simulink model "MAE547Project_part5ModifiedToWorkWithSingularity"  (R2020b)
settings: Solver=VariableStepAuto  StartTime=0.0  StopTime=5  RelTol=1e-3
values from neighbouring files (symbols this model uses):
  Arm = dhfunc(descriptor,d,a,alpha,theta,m,I,r,G,Jm,fv)    [Test.m]    (also in TestZone.m = dhfunc(descriptor,d,a,alpha,theta,m,I,r,G,Jm, Fv); TestZone2.m = dhfunc(descriptor,d,a,alpha,theta,m,I,r,G,Jm, Fc, Fv); TestZone2WithSingularity.m = dhfunc(descriptor,d,a,alpha,theta,m,I,r,G,Jm, Fv); dhfunc.m = SerialLink(LinkList, 'name', 'Arm'))
  ddod = [0; 0; 0]    [TestZone2.m]    (also in TestZone2WithSingularity.m)
  ddq = [0,0,0,0,0,0]    [TestZone2WithSingularity.m]
  dod = [0; 0; 0]    [TestZone2.m]    (also in TestZone2WithSingularity.m)
  dqIntial = [0, 0, 0]    [TestZone2.m]    (also in TestZone2WithSingularity.m = [0,0,0,0,0,0])
  dwd = [0; 0; 0]    [TestZone2.m]    (also in TestZone2WithSingularity.m)
  heIntial = [0;0;0;0;0;0]    [TestZone2.m]    (also in TestZone2WithSingularity.m)
  Kd = eye(6)*kd    [TestZone.m]    (also in TestZone2.m = eye(3)*kd; TestZone2WithSingularity.m; Workspace.mat = [1 0 0 0 0 0 0 1 0 0 0 0 ... (36 elements, 6x6)])
  Kp = eye(6)*kp    [TestZone.m]    (also in TestZone2.m = eye(3)*kp; TestZone2WithSingularity.m; Workspace.mat = [1 0 0 0 0 0 0 1 0 0 0 0 ... (36 elements, 6x6)])
  ksingle = 0.5    [TestZone2WithSingularity.m]
  Md = eye(3)*md    [TestZone2.m]    (also in TestZone2WithSingularity.m = eye(6)*md)
  od = [1;2;1]    [TestZone2.m]    (also in TestZone2WithSingularity.m = [4; 1; 5])
  qIntial = [0,0,0]    [TestZone2.m]    (also in TestZone2WithSingularity.m = [1,0,1,0,1,0])
  Rd = [1 0 0; 0 1 0; 0 0 1]    [TestZone2.m]    (also in TestZone2WithSingularity.m = [0.9364 -0.2667 -0.2281; 0.1622 -0.2476 0.9552  ;-0.3112 -0.)
  wd = [0; 0; 0]    [TestZone2.m]    (also in TestZone2WithSingularity.m)
libraries: roblocks x1
settings Model: Creator=Runa Nakamura  LastModifiedBy=kylej
settings DebuggingCC: AlgebraicLoopMsg=none

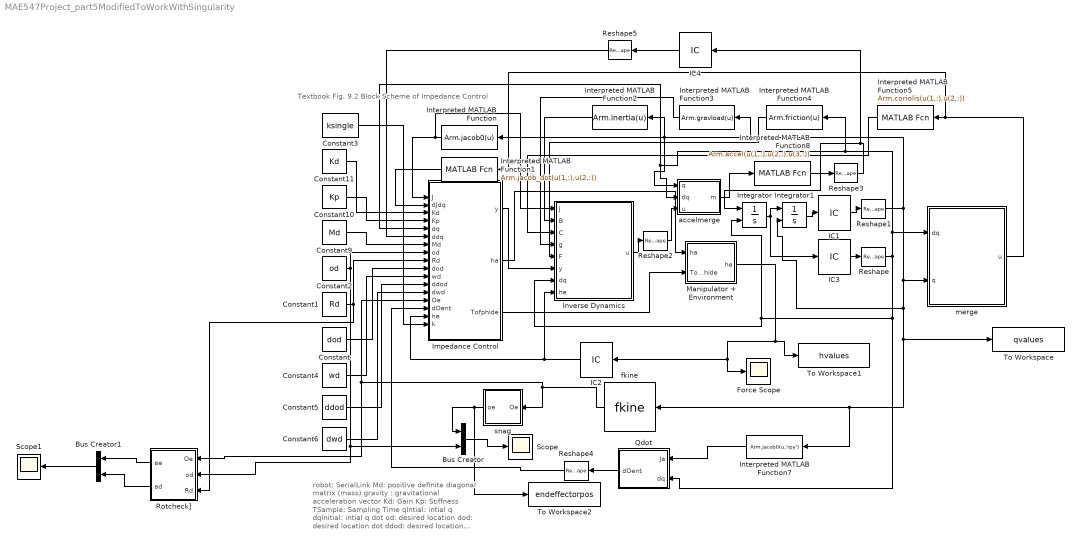
== system MAE547Project_part5ModifiedToWorkWithSingularity ==
  note: robot: SerialLink
      | Md: positive definite diagonal matrix (mass)
      | gravity : gravitational acceleration vector
      | Kd: Gain
      | Kp: Stiffness
      | TSample: Sampling Time
      | qIntial: intial q
      | dqInitial: intial q dot
      | od: desired location
      | dod: desired location dot
      | ddod: desired location double dot
      | Rd: desired orientation
      | wd: desired orientation dot
      | dwd: desired orientation double dot
      | heIntial: intial he value
  note: Textbook Fig. 9.2 Block Scheme of Impedance Control
  Bus Creator : BusCreator  Inputs=2
  Bus Creator1 : BusCreator  Inputs=2
  Constant : Constant  Value=dod
  Constant1 : Constant  Value=Rd
  Constant10 : Constant  Value=Kp
  Constant11 : Constant  Value=Kd
  Constant2 : Constant  Value=od
  Constant3 : Constant  Value=ksingle
  Constant4 : Constant  Value=wd
  Constant5 : Constant  Value=ddod
  Constant6 : Constant  Value=dwd
  Constant9 : Constant  Value=Md
  Force Scope : Scope
  IC1 : InitialCondition  Value=qIntial
  IC2 : InitialCondition  Value=heIntial
  IC3 : InitialCondition  Value=dqIntial
  IC4 : InitialCondition  Value=ddq
  Impedance Control : MATLAB Function  TreatAsAtomicUnit=on
  Integrator : Integrator  InitialConditionSource=external  ZeroCross=off
  Integrator1 : Integrator  InitialConditionSource=external  ZeroCross=off
  Interpreted MATLAB Function : MATLABFcn  MATLABFcn=Arm.jacob0(u)  Output1D=off
  Interpreted MATLAB Function1 : MATLABFcn  MATLABFcn=Arm.jacob_dot(u(1,:),u(2,:))  Output1D=off
  Interpreted MATLAB Function2 : MATLABFcn  MATLABFcn=Arm.inertia(u)  Output1D=off
  Interpreted MATLAB Function3 : MATLABFcn  MATLABFcn=Arm.gravload(u)  Output1D=off
  Interpreted MATLAB Function4 : MATLABFcn  MATLABFcn=Arm.friction(u)  Output1D=off
  Interpreted MATLAB Function5 : MATLABFcn  MATLABFcn=Arm.coriolis(u(1,:),u(2,:))  Output1D=off
  Interpreted MATLAB Function7 : MATLABFcn  MATLABFcn=Arm.jacob0(u,'rpy')  Output1D=off
  Interpreted MATLAB Function8 : MATLABFcn  MATLABFcn=Arm.accel(u(1,:),u(2,:),u(3,:))  Output1D=off
  Inverse Dynamics : MATLAB Function  TreatAsAtomicUnit=on
  Manipulator + Environment : MATLAB Function  TreatAsAtomicUnit=on
  Qdot : MATLAB Function  TreatAsAtomicUnit=on
  Reshape{,1..5} (6 alike) : Reshape  OutputDimensionality=Row vector (2-D)
  Rotcheck] : MATLAB Function  TreatAsAtomicUnit=on
  Scope : Scope
  Scope1 : Scope
  To Workspace : ToWorkspace  VariableName=qvalues  SaveFormat=Timeseries  SampleTime=-1
  To Workspace1 : ToWorkspace  VariableName=hvalues  SaveFormat=Timeseries  SampleTime=-1
  To Workspace2 : ToWorkspace  VariableName=endeffectorpos  SaveFormat=Timeseries  SampleTime=-1
  accelmerge : MATLAB Function  TreatAsAtomicUnit=on
  fkine : roblocks/Arm/fkine  robot=Arm
  merge : MATLAB Function  TreatAsAtomicUnit=on
  snag : MATLAB Function  TreatAsAtomicUnit=on
  wires:
  Impedance Control/1(y) -> Inverse Dynamics/6(y)
  fkine/1 -> snag/1(Oe), Rotcheck]/1(Oe), Impedance Control/14(Oe)
  Constant2/1 -> Rotcheck]/2(od), Bus Creator/2, Impedance Control/8(od)
  Constant1/1 -> Rotcheck]/3(Rd), Impedance Control/9(Rd)
  Constant/1 -> Impedance Control/10(dod)
  Constant4/1 -> Impedance Control/11(wd)
  Constant5/1 -> Impedance Control/12(ddod)
  Constant6/1 -> Impedance Control/13(dwd)
  Constant9/1 -> Impedance Control/7(Md)
  Constant11/1 -> Impedance Control/3(Kd)
  Constant10/1 -> Impedance Control/4(Kp)
  Reshape/1 -> merge/1(dq), Interpreted MATLAB Function4/1, accelmerge/2(dq), Impedance Control/5(dq), Qdot/2(dq), Integrator/2, Inverse Dynamics/7(dq)
  IC2/1 -> Inverse Dynamics/8(he), Impedance Control/16(he)
  Manipulator + Environment/1(he) -> IC2/1, Force Scope/1, To Workspace1/1
  Impedance Control/3(Tofphide) -> Manipulator + Environment/2(Tofphide)
  Impedance Control/2(ha) -> Manipulator + Environment/1(ha)
  Interpreted MATLAB Function/1 -> Inverse Dynamics/1(J), Impedance Control/1(J)
  Interpreted MATLAB Function1/1 -> Impedance Control/2(dJdq)
  Interpreted MATLAB Function2/1 -> Inverse Dynamics/2(B)
  Interpreted MATLAB Function3/1 -> Inverse Dynamics/4(g)
  Interpreted MATLAB Function4/1 -> Inverse Dynamics/5(F)
  merge/1(u) -> Interpreted MATLAB Function1/1, Interpreted MATLAB Function5/1
  Interpreted MATLAB Function5/1 -> Inverse Dynamics/3(C)
  Qdot/1(dOent) -> Reshape4/1
  IC3/1 -> Reshape/1
  IC1/1 -> Reshape1/1
  accelmerge/1(m) -> Interpreted MATLAB Function8/1
  Integrator/1 -> Integrator1/1, IC3/1
  Integrator1/1 -> IC1/1
  Inverse Dynamics/1(u) -> Reshape2/1
  Reshape2/1 -> accelmerge/3(u)
  Interpreted MATLAB Function8/1 -> Reshape3/1
  Reshape3/1 -> IC4/1, Integrator/1
  Bus Creator/1 -> Scope/1
  Reshape1/1 -> Interpreted MATLAB Function2/1, Interpreted MATLAB Function/1, accelmerge/1(q), Interpreted MATLAB Function3/1, To Workspace/1, fkine/1, Interpreted MATLAB Function7/1, Integrator1/2, merge/2(q)
  snag/1(oe) -> Bus Creator/1, To Workspace2/1
  Constant3/1 -> Impedance Control/17(k)
  Bus Creator1/1 -> Scope1/1
  Rotcheck]/2(ad) -> Bus Creator1/2
  Rotcheck]/1(ae) -> Bus Creator1/1
  Interpreted MATLAB Function7/1 -> Qdot/1(Ja)
  Reshape4/1 -> Impedance Control/15(dOent)
  IC4/1 -> Reshape5/1
  Reshape5/1 -> Impedance Control/6(ddq)

== matlab function MAE547Project_part5ModifiedToWorkWithSingularity/Rotcheck] ==
  data: Oe input; ae output; od input; ad output; Rd input
function [ae,ad]  = RotCheck(Oe,od,Rd)
Od =[Rd od; 0 0 0 1];
ae = tform2eul(Oe);
ad = tform2eul(Od);
end

== matlab function MAE547Project_part5ModifiedToWorkWithSingularity/Inverse Dynamics ==
  data: J input; B input; C input; g input; F input; y input; u output; dq input; he input
function u  = InverseD(J,B,C,g,F,y,dq,he)
dq = dq';

F = diag(F);
n = C*dq+F*dq+g';            %(8.56 Textbook)
u = B*y+n+J'*he;           %(9.30 Textbook)

== matlab function MAE547Project_part5ModifiedToWorkWithSingularity/Impedance Control ==
  data: J input; dJdq input; Kd input; Kp input; dq input; ddq input; Md input; od input; Rd input; dod input; wd input; y output; ddod input; dwd input; Oe input; dOent input; he input; ha output; Tofphide output; k input
function [y,ha,Tofphide] = ImpedC(J,dJdq,Kd,Kp,dq,ddq,Md,od,Rd,dod,wd,ddod,dwd,Oe,dOent,he,k)        %Corke
Od = [Rd od ; 0 0 0 1]; %Making the capital O desired

dq = dq';

Te = Oe; %These are from the equation above 9.8 in the book just
Td = Od; %Just using these lines to maintain notation 

Rtd = Td(1:3,1:3).'; %Grabbing transpose of desired rotation for use later

Tde = inv(Td)*Te; %9.8 from the book

odde = Tde(1:3, 4); %3x1 vector of the postions 
wdd = Rtd*wd; %Grabbing wdd
Tofphide = Tde(1:3,1:3); %Snaging The rotation matrix for ease of use later

Jad = inv([eye(3), zeros(3); zeros(3), Tofphide])*[Rtd, zeros(3); zeros(3), Rtd] *J;

%Repeating for Jdotad

dwdd = Rtd*dwd; %Grabbing dwdd

S = zeros(3);
dS = zeros(3);
S = skew(wdd); %3.9
dodde = Rtd*(dOent(1:3)'-dod) - S*(Rtd*(Oe(1:3, 4) - od));
dphide = inv(Tofphide)*Rtd*(dOent(4:6)'-wd);
dTofphide = eul2rotm(dphide');

%Grabbing a Jad Dot
dJaddq = inv([eye(3), zeros(3); zeros(3), dTofphide])*[Rtd, zeros(3); zeros(3), Rtd] *dJdq;



%Finding dS
dS = skew(dwdd);
%Finding b matrix
b = [Rtd*dod+S*odde; inv(Tofphide)*wdd]; %near (9.34)

%Finding db
db = [Rtd*ddod + dS*dodde; inv(dTofphide)*dwdd]; %near (9.34)


phide = tform2eul(Tde,'XYZ'); %euler transformation using corke

sx = -[odde; phide']; %eq

ha = Kp*sx; %From notes

dsx = -Jad*dq+b;     %(9.33 textbook)

ddsx = -Jad*ddq' - dJaddq + db;


Icustom = eye(length(Jad(:,1)));
invJad = Jad'*inv(Jad*Jad'+k^2*Icustom);
hde = [0,0,0,0,0,0]'; %NEED TO FIX
y = invJad*inv(Md)*(Kd*dsx+Kp*sx-Md*dJaddq+Md*db-hde); %9.35

== matlab function MAE547Project_part5ModifiedToWorkWithSingularity/Manipulator + Environment ==
  data: he output; ha input; Tofphide input
function he = ME(ha,Tofphide)
% he = inv(Tofphide)*ha;
he = inv([eye(3), zeros(3); zeros(3), Tofphide])*ha;
end

== matlab function MAE547Project_part5ModifiedToWorkWithSingularity/accelmerge ==
  data: m output; q input; dq input; u input
function m = m(q, dq, u)
% he = inv(Tofphide)*ha;
m = [q;dq;u];
end

== matlab function MAE547Project_part5ModifiedToWorkWithSingularity/merge ==
  data: dq input; q input; u output
function u  = merge(dq,q)
u = [q;dq];

== matlab function MAE547Project_part5ModifiedToWorkWithSingularity/snag ==
  data: Oe input; oe output
function oe  = snag(Oe)
oe = Oe(1:3,4);
end

== matlab function MAE547Project_part5ModifiedToWorkWithSingularity/Qdot ==
  data: dOent output; Ja input; dq input
function dOent = ME(Ja,dq)
dOent = Ja*dq';
end
